simulink model "first"  (R2023b)
settings: Solver=VariableStepAuto  StartTime=0.0  StopTime=10.0  RelTol=1e-3
libraries: arduinolib x13, arduinosensorlib x4
settings Model: Creator=tjrgu  LastModifiedBy=tjrgu

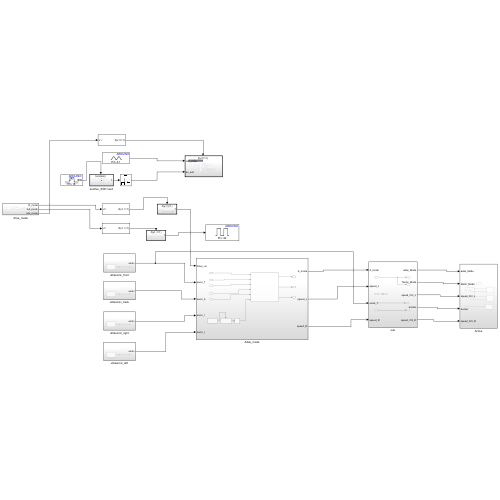
[thumbnail: Simulink's stored preview of the top-level diagram]
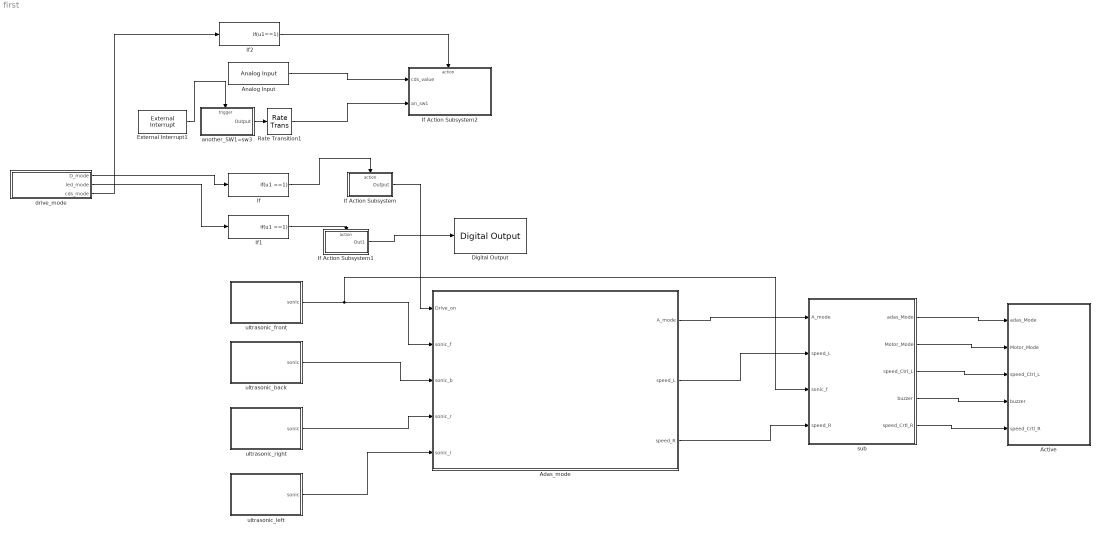
== system first ==
  Active : Subsystem
  Adas_mode : Subsystem
  Analog Input : arduinolib/Analog Input  pinNumber=1  ReadResultsOnly=off  ConversionTriggerSource=Software  ExternalTriggerType=uint32( 0 )  OutputDataType=uint16  EnableConversionCompleteNotify=off  EnableOuputStatus=off  SampleTime=-1  blockPlatform=arduino
  Digital Output : arduinolib/Digital Output  pinNumber=42  Direction=output  blockPlatform=arduino
  External Interrupt1 : arduinolib/External Interrupt  Pin=18  PullUp=off  Mode=RISING  InterruptSimulationInput=off
  If : If  IfExpression=u1 ==1  ShowElse=off
  If Action Subsystem : Subsystem  TreatAsAtomicUnit=on
  If Action Subsystem1 : Subsystem  TreatAsAtomicUnit=on
  If Action Subsystem2 : Subsystem  TreatAsAtomicUnit=on
  If1 : If  IfExpression=u1 ==1  ShowElse=off
  If2 : If  IfExpression=u1==1  ShowElse=off
  Rate Transition1 : RateTransition  Integrity=off
  another_SW1=sw3 : Subsystem
  drive_mode : Subsystem
  sub : Subsystem
  ultrasonic_back : Subsystem
  ultrasonic_front : Subsystem
  ultrasonic_left : Subsystem
  ultrasonic_right : Subsystem
  wires:
  ultrasonic_front/1(sonic) -> sub/3(sonic_f), Adas_mode/2(sonic_f)
  drive_mode/1(D_mode) -> If/1
  ultrasonic_back/1(sonic) -> Adas_mode/3(sonic_b)
  ultrasonic_right/1(sonic) -> Adas_mode/4(sonic_r)
  ultrasonic_left/1(sonic) -> Adas_mode/5(sonic_l)
  Adas_mode/1(A_mode) -> sub/1(A_mode)
  Adas_mode/2(speed_L) -> sub/2(speed_L)
  Adas_mode/3(speed_R) -> sub/4(speed_R)
  sub/1(adas_Mode) -> Active/1(adas_Mode)
  sub/2(Motor_Mode) -> Active/2(Motor_Mode)
  sub/3(speed_Ctrl_L) -> Active/3(speed_Ctrl_L)
  sub/4(buzzer) -> Active/4(buzzer)
  sub/5(speed_Crtl_R) -> Active/5(speed_Crtl_R)
  If/1 -> If Action Subsystem/Action
  If Action Subsystem/1(Output) -> Adas_mode/1(Drive_on)
  drive_mode/2(led_mode) -> If1/1
  If1/1 -> If Action Subsystem1/Action
  If Action Subsystem1/1(Out1) -> Digital Output/1
  drive_mode/3(cds_mode) -> If2/1
  If2/1 -> If Action Subsystem2/Action
  Analog Input/1 -> If Action Subsystem2/1(cds_value)
  External Interrupt1/1 -> another_SW1=sw3/Trigger
  another_SW1=sw3/1(Output) -> Rate Transition1/1
  Rate Transition1/1 -> If Action Subsystem2/2(an_sw1)

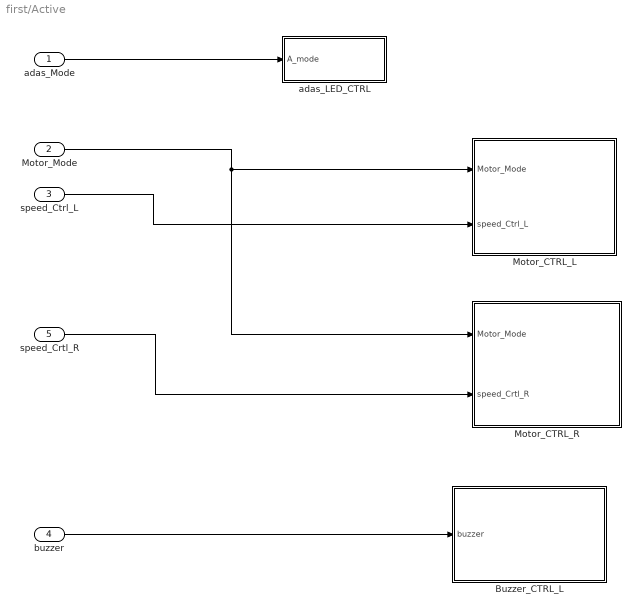
== system first/Active ==
  adas_Mode : Inport
  Motor_Mode : Inport  Port=2
  speed_Ctrl_L : Inport  Port=3
  buzzer : Inport  Port=4
  speed_Crtl_R : Inport  Port=5
  Buzzer_CTRL_L : Subsystem
  Motor_CTRL_L : Subsystem
  Motor_CTRL_R : Subsystem
  adas_LED_CTRL : Subsystem
  wires:
  Motor_Mode/1 -> Motor_CTRL_R/1(Motor_Mode), Motor_CTRL_L/1(Motor_Mode)
  speed_Ctrl_L/1 -> Motor_CTRL_L/2(speed_Ctrl_L)
  speed_Crtl_R/1 -> Motor_CTRL_R/2(speed_Crtl_R)
  buzzer/1 -> Buzzer_CTRL_L/1(buzzer)
  adas_Mode/1 -> adas_LED_CTRL/1(A_mode)

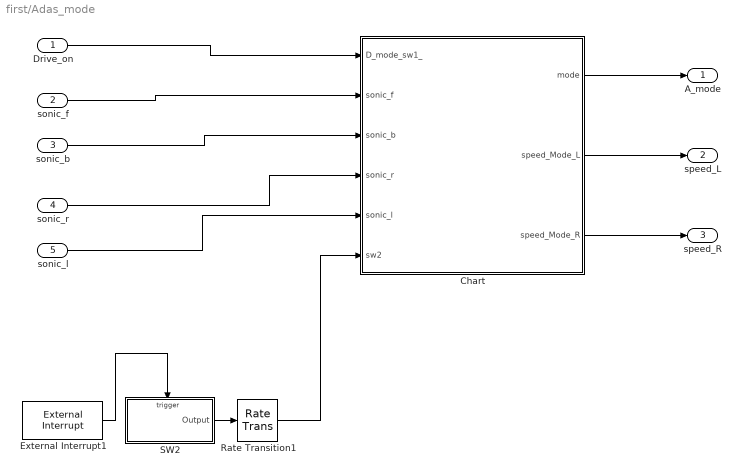
== system first/Adas_mode ==
  Drive_on : Inport
  sonic_f : Inport  Port=2
  sonic_b : Inport  Port=3
  sonic_r : Inport  Port=4
  sonic_l : Inport  Port=5
  Chart : Stateflow chart  TreatAsAtomicUnit=on
  External Interrupt1 : arduinolib/External Interrupt  Pin=3  PullUp=off  Mode=RISING  InterruptSimulationInput=off
  Rate Transition1 : RateTransition  Integrity=off
  SW2 : Subsystem
  A_mode : Outport
  speed_L : Outport  Port=2
  speed_R : Outport  Port=3
  wires:
  sonic_f/1 -> Chart/2(sonic_f)
  External Interrupt1/1 -> SW2/Trigger
  SW2/1(Output) -> Rate Transition1/1
  Rate Transition1/1 -> Chart/6(sw2)
  Drive_on/1 -> Chart/1(D_mode_sw1_)
  sonic_b/1 -> Chart/3(sonic_b)
  sonic_r/1 -> Chart/4(sonic_r)
  sonic_l/1 -> Chart/5(sonic_l)
  Chart/1(mode) -> A_mode/1
  Chart/2(speed_Mode_L) -> speed_L/1
  Chart/3(speed_Mode_R) -> speed_R/1

== system first/If Action Subsystem ==
  Action Port : ActionPort  ActionPortLabel=if(u1 ==1)
  Constant : Constant
  Output : Outport
  wires:
  Constant/1 -> Output/1

== system first/If Action Subsystem1 ==
  Action Port : ActionPort  ActionPortLabel=if(u1 ==1)
  Constant : Constant
  Out1 : Outport
  wires:
  Constant/1 -> Out1/1

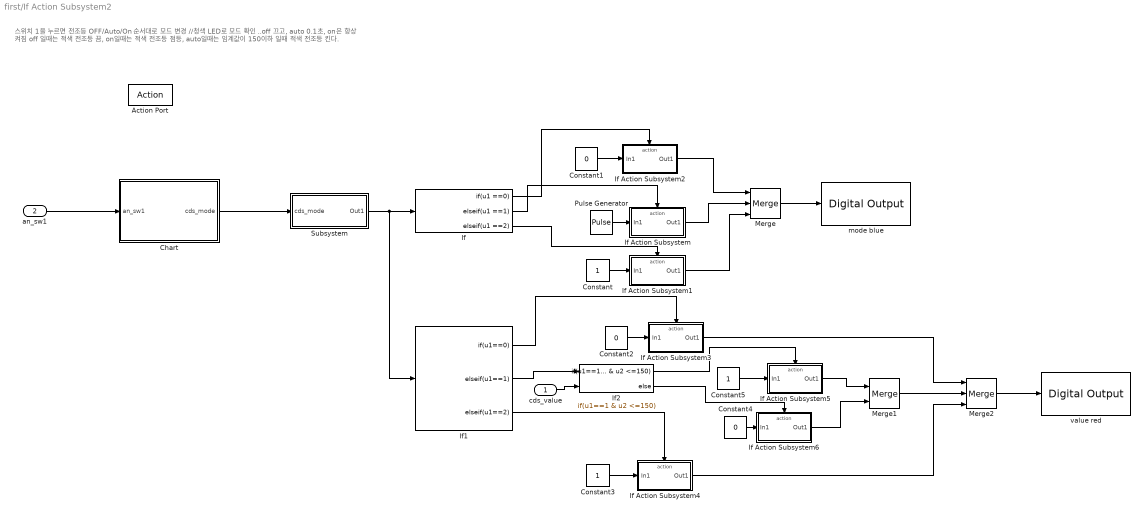
== system first/If Action Subsystem2 ==
  note: 스위치 1을  누르면 전조등 OFF/Auto/On 순서대로 모드 변경 //청색 LED로 모드 확인 ..off 끄고, auto 0.1초, on은 항상 켜짐
      | off 일때는 적색 전조등 끔, on일때는 적색 전조등 점등, auto일때는 임계값이 150이하 일때 적색 전조등 킨다.
  cds_value : Inport
  an_sw1 : Inport  Port=2
  Action Port : ActionPort  ActionPortLabel=if(u1==1)
  Chart : Stateflow chart  TreatAsAtomicUnit=on
  Constant : Constant
  Constant1 : Constant  Value=0
  Constant2 : Constant  Value=0
  Constant3 : Constant
  Constant4 : Constant  Value=0
  Constant5 : Constant
  If : If  IfExpression=u1 ==0  ElseIfExpressions=u1 ==1,u1 ==2  ShowElse=off
  If Action Subsystem : Subsystem  TreatAsAtomicUnit=on
  If Action Subsystem1 : Subsystem  TreatAsAtomicUnit=on
  If Action Subsystem2 : Subsystem  TreatAsAtomicUnit=on
  If Action Subsystem3 : Subsystem  TreatAsAtomicUnit=on
  If Action Subsystem4 : Subsystem  TreatAsAtomicUnit=on
  If Action Subsystem5 : Subsystem  TreatAsAtomicUnit=on
  If Action Subsystem6 : Subsystem  TreatAsAtomicUnit=on
  If1 : If  IfExpression=u1==0  ElseIfExpressions=u1==1, u1==2  ShowElse=off
  If2 : If  NumInputs=2  IfExpression=u1==1 & u2 <=150
  Merge : Merge  Inputs=3
  Merge1 : Merge
  Merge2 : Merge  Inputs=3
  Pulse Generator : DiscretePulseGenerator  PulseType=Time based  Period=0.2  PulseWidth=50
  Subsystem : Subsystem
  mode blue : arduinolib/Digital Output  pinNumber=45  Direction=output  blockPlatform=arduino
  value red : arduinolib/Digital Output  pinNumber=44  Direction=output  blockPlatform=arduino
  wires:
  an_sw1/1 -> Chart/1(an_sw1)
  Chart/1(cds_mode) -> Subsystem/1(cds_mode)
  Subsystem/1(Out1) -> If1/1, If/1
  If/2 -> If Action Subsystem/Action
  Pulse Generator/1 -> If Action Subsystem/1(In1)
  If/3 -> If Action Subsystem1/Action
  Constant/1 -> If Action Subsystem1/1(In1)
  If/1 -> If Action Subsystem2/Action
  Constant1/1 -> If Action Subsystem2/1(In1)
  If Action Subsystem2/1(Out1) -> Merge/1
  If Action Subsystem/1(Out1) -> Merge/2
  If Action Subsystem1/1(Out1) -> Merge/3
  Merge/1 -> mode blue/1
  If1/1 -> If Action Subsystem3/Action
  Constant2/1 -> If Action Subsystem3/1(In1)
  If1/3 -> If Action Subsystem4/Action
  Constant3/1 -> If Action Subsystem4/1(In1)
  If1/2 -> If2/1
  cds_value/1 -> If2/2
  If2/1 -> If Action Subsystem5/Action
  If2/2 -> If Action Subsystem6/Action
  Constant4/1 -> If Action Subsystem6/1(In1)
  Constant5/1 -> If Action Subsystem5/1(In1)
  If Action Subsystem5/1(Out1) -> Merge1/1
  If Action Subsystem6/1(Out1) -> Merge1/2
  If Action Subsystem3/1(Out1) -> Merge2/1
  Merge1/1 -> Merge2/2
  If Action Subsystem4/1(Out1) -> Merge2/3
  Merge2/1 -> value red/1

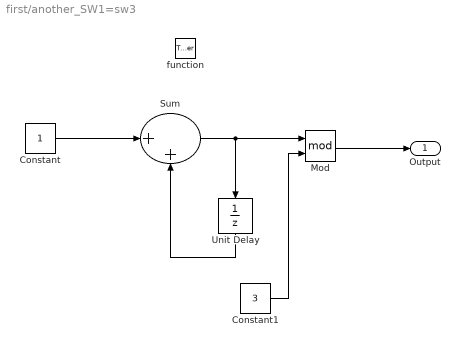
== system first/another_SW1=sw3 ==
  function : TriggerPort  TriggerType=function-call  VariantControl=(inherit)
  Constant : Constant
  Constant1 : Constant  Value=3
  Mod : Math  Operator=mod
  Sum : Sum  Inputs=|++
  Unit Delay : UnitDelay  SampleTime=-1  HasFrameUpgradeWarning=on
  Output : Outport
  wires:
  Constant/1 -> Sum/1
  Sum/1 -> Unit Delay/1, Mod/1
  Constant1/1 -> Mod/2
  Unit Delay/1 -> Sum/2
  Mod/1 -> Output/1

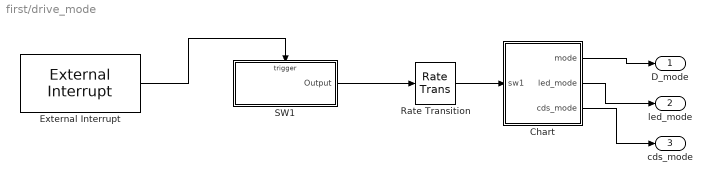
== system first/drive_mode ==
  Chart : Stateflow chart  TreatAsAtomicUnit=on
  External Interrupt : arduinolib/External Interrupt  Pin=2  PullUp=off  Mode=RISING  InterruptSimulationInput=off
  Rate Transition : RateTransition  Integrity=off
  SW1 : Subsystem
  D_mode : Outport
  led_mode : Outport  Port=2
  cds_mode : Outport  Port=3
  wires:
  External Interrupt/1 -> SW1/Trigger
  SW1/1(Output) -> Rate Transition/1
  Rate Transition/1 -> Chart/1(sw1)
  Chart/1(mode) -> D_mode/1
  Chart/2(led_mode) -> led_mode/1
  Chart/3(cds_mode) -> cds_mode/1

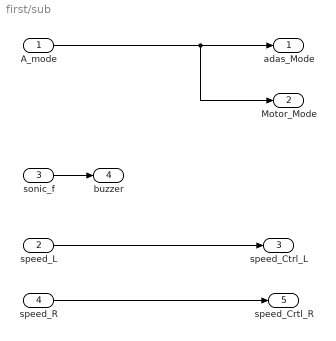
== system first/sub ==
  A_mode : Inport
  speed_L : Inport  Port=2
  sonic_f : Inport  Port=3
  speed_R : Inport  Port=4
  adas_Mode : Outport
  Motor_Mode : Outport  Port=2
  speed_Ctrl_L : Outport  Port=3
  buzzer : Outport  Port=4
  speed_Crtl_R : Outport  Port=5
  wires:
  A_mode/1 -> Motor_Mode/1, adas_Mode/1
  speed_L/1 -> speed_Ctrl_L/1
  speed_R/1 -> speed_Crtl_R/1
  sonic_f/1 -> buzzer/1

== system first/ultrasonic_back ==
  note: 초음파 계수 10
      | 실제 요구사항 : 50cm , 10cm
      | 변경 요구사항 : 초음파값 5,1
  Gain : Gain  Gain=10
  Ultrasonic Sensor : arduinosensorlib/Ultrasonic Sensor  NumSignalPins=2  TrigPin=48  EchoPin=49  SignalPin=3  SampleTime_=0.1  blockPlatform=ARDUINO
  sonic : Outport
  wires:
  Ultrasonic Sensor/1 -> Gain/1
  Gain/1 -> sonic/1

== system first/ultrasonic_front ==
  note: 초음파 계수 10
      | 실제 요구사항 : 50cm , 10cm
      | 변경 요구사항 : 초음파값 5,1
  Gain : Gain  Gain=10
  Ultrasonic Sensor : arduinosensorlib/Ultrasonic Sensor  NumSignalPins=2  TrigPin=46  EchoPin=47  SignalPin=3  SampleTime_=0.1  blockPlatform=ARDUINO
  sonic : Outport
  wires:
  Ultrasonic Sensor/1 -> Gain/1
  Gain/1 -> sonic/1

== system first/ultrasonic_left ==
  note: 초음파 계수 10
      | 실제 요구사항 : 50cm , 10cm
      | 변경 요구사항 : 초음파값 5,1
  Gain : Gain  Gain=10
  Ultrasonic Sensor : arduinosensorlib/Ultrasonic Sensor  NumSignalPins=2  TrigPin=52  EchoPin=53  SignalPin=3  SampleTime_=0.1  blockPlatform=ARDUINO
  sonic : Outport
  wires:
  Ultrasonic Sensor/1 -> Gain/1
  Gain/1 -> sonic/1

== system first/ultrasonic_right ==
  note: 초음파 계수 10
      | 실제 요구사항 : 50cm , 10cm
      | 변경 요구사항 : 초음파값 5,1
  Gain : Gain  Gain=10
  Ultrasonic Sensor : arduinosensorlib/Ultrasonic Sensor  NumSignalPins=2  TrigPin=50  EchoPin=51  SignalPin=3  SampleTime_=0.1  blockPlatform=ARDUINO
  sonic : Outport
  wires:
  Ultrasonic Sensor/1 -> Gain/1
  Gain/1 -> sonic/1

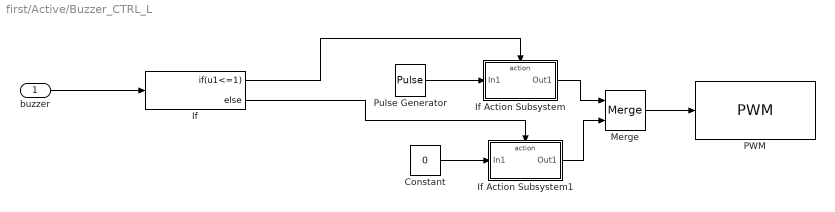
== system first/Active/Buzzer_CTRL_L ==
  buzzer : Inport
  Constant : Constant  Value=0
  If : If  IfExpression=u1<=1
  If Action Subsystem : Subsystem  TreatAsAtomicUnit=on
  If Action Subsystem1 : Subsystem  TreatAsAtomicUnit=on
  Merge : Merge
  PWM : arduinolib/PWM  pinNumber=4  frequencyType=Default  desiredFrequency=490.2  achievableFrequency=490.2
  Pulse Generator : DiscretePulseGenerator  PulseType=Time based  Period=0.4  PulseWidth=50
  wires:
  buzzer/1 -> If/1
  Pulse Generator/1 -> If Action Subsystem/1(In1)
  If/2 -> If Action Subsystem1/Action
  Constant/1 -> If Action Subsystem1/1(In1)
  If Action Subsystem/1(Out1) -> Merge/1
  If Action Subsystem1/1(Out1) -> Merge/2
  Merge/1 -> PWM/1
  If/1 -> If Action Subsystem/Action

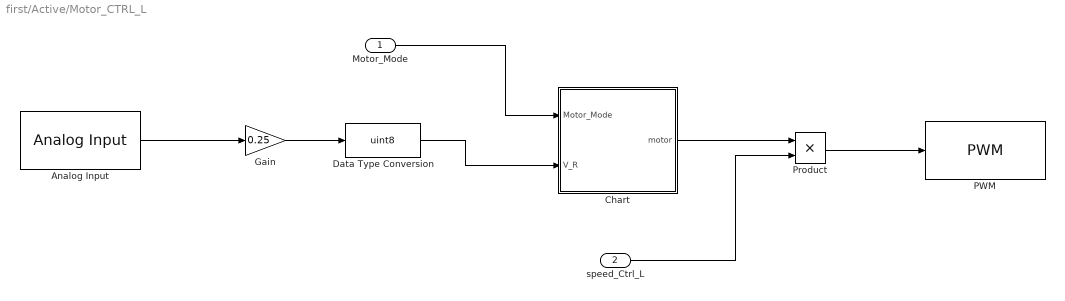
== system first/Active/Motor_CTRL_L ==
  Motor_Mode : Inport
  speed_Ctrl_L : Inport  Port=2
  Analog Input : arduinolib/Analog Input  pinNumber=0  ReadResultsOnly=off  ConversionTriggerSource=Software  ExternalTriggerType=uint32( 0 )  OutputDataType=uint16  EnableConversionCompleteNotify=off  EnableOuputStatus=off  SampleTime=-1  blockPlatform=arduino
  Chart : Stateflow chart  TreatAsAtomicUnit=on
  Data Type Conversion : DataTypeConversion  OutDataTypeStr=uint8  SaturateOnIntegerOverflow=off  RndMeth=Floor
  Gain : Gain  Gain=0.25
  PWM : arduinolib/PWM  pinNumber=11  frequencyType=Default  desiredFrequency=490.2  achievableFrequency=490.2
  Product : Product
  wires:
  Analog Input/1 -> Gain/1
  Gain/1 -> Data Type Conversion/1
  Motor_Mode/1 -> Chart/1(Motor_Mode)
  Data Type Conversion/1 -> Chart/2(V_R)
  Chart/1(motor) -> Product/1
  speed_Ctrl_L/1 -> Product/2
  Product/1 -> PWM/1

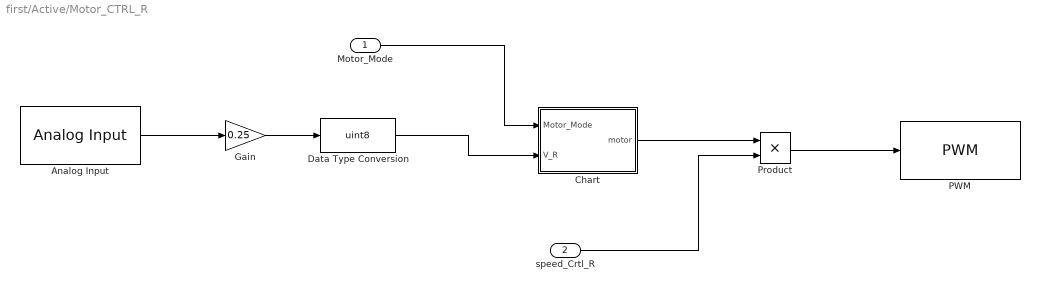
== system first/Active/Motor_CTRL_R ==
  Motor_Mode : Inport
  speed_Crtl_R : Inport  Port=2
  Analog Input : arduinolib/Analog Input  pinNumber=0  ReadResultsOnly=off  ConversionTriggerSource=Software  ExternalTriggerType=uint32( 0 )  OutputDataType=uint16  EnableConversionCompleteNotify=off  EnableOuputStatus=off  SampleTime=-1  blockPlatform=arduino
  Chart : Stateflow chart  TreatAsAtomicUnit=on
  Data Type Conversion : DataTypeConversion  OutDataTypeStr=uint8  SaturateOnIntegerOverflow=off  RndMeth=Floor
  Gain : Gain  Gain=0.25
  PWM : arduinolib/PWM  pinNumber=3  frequencyType=Default  desiredFrequency=490.2  achievableFrequency=490.2
  Product : Product
  wires:
  Gain/1 -> Data Type Conversion/1
  Analog Input/1 -> Gain/1
  Motor_Mode/1 -> Chart/1(Motor_Mode)
  Data Type Conversion/1 -> Chart/2(V_R)
  Chart/1(motor) -> Product/1
  speed_Crtl_R/1 -> Product/2
  Product/1 -> PWM/1

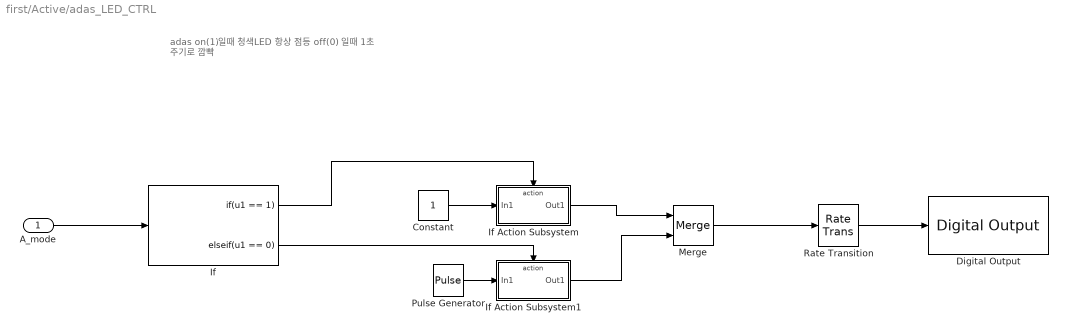
== system first/Active/adas_LED_CTRL ==
  note: adas on(1)일때 청색LED 항상 점등
      | off(0) 일때 1초 주기로 깜빡
  A_mode : Inport
  Constant : Constant
  Digital Output : arduinolib/Digital Output  pinNumber=43  Direction=output  blockPlatform=arduino
  If : If  IfExpression=u1 == 1  ElseIfExpressions=u1 == 0  ShowElse=off
  If Action Subsystem : Subsystem  TreatAsAtomicUnit=on
  If Action Subsystem1 : Subsystem  TreatAsAtomicUnit=on
  Merge : Merge
  Pulse Generator : DiscretePulseGenerator  PulseType=Time based  PulseWidth=50
  Rate Transition : RateTransition  Integrity=off
  wires:
  A_mode/1 -> If/1
  If/1 -> If Action Subsystem/Action
  Constant/1 -> If Action Subsystem/1(In1)
  If/2 -> If Action Subsystem1/Action
  Pulse Generator/1 -> If Action Subsystem1/1(In1)
  If Action Subsystem/1(Out1) -> Merge/1
  If Action Subsystem1/1(Out1) -> Merge/2
  Merge/1 -> Rate Transition/1
  Rate Transition/1 -> Digital Output/1

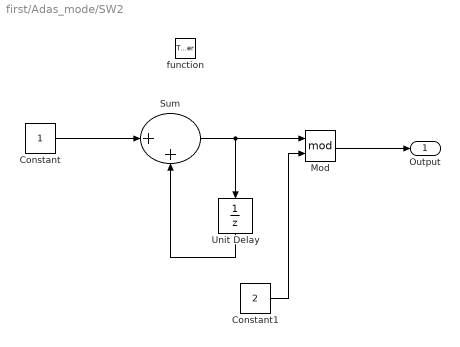
== system first/Adas_mode/SW2 ==
  function : TriggerPort  TriggerType=function-call  VariantControl=(inherit)
  Constant : Constant
  Constant1 : Constant  Value=2
  Mod : Math  Operator=mod
  Sum : Sum  Inputs=|++
  Unit Delay : UnitDelay  SampleTime=-1  HasFrameUpgradeWarning=on
  Output : Outport
  wires:
  Constant/1 -> Sum/1
  Sum/1 -> Unit Delay/1, Mod/1
  Constant1/1 -> Mod/2
  Unit Delay/1 -> Sum/2
  Mod/1 -> Output/1

== system first/If Action Subsystem2/If Action Subsystem ==
  In1 : Inport
  Action Port : ActionPort  ActionPortLabel=elseif(u1 ==1)
  Out1 : Outport
  wires:
  In1/1 -> Out1/1

== system first/If Action Subsystem2/If Action Subsystem1 ==
  In1 : Inport
  Action Port : ActionPort  ActionPortLabel=elseif(u1 ==2)
  Out1 : Outport
  wires:
  In1/1 -> Out1/1

== system first/If Action Subsystem2/If Action Subsystem2 ==
  In1 : Inport
  Action Port : ActionPort  ActionPortLabel=if(u1 ==0)
  Out1 : Outport
  wires:
  In1/1 -> Out1/1

== system first/If Action Subsystem2/If Action Subsystem3 ==
  In1 : Inport
  Action Port : ActionPort  ActionPortLabel=if(u1==0)
  Out1 : Outport
  wires:
  In1/1 -> Out1/1

== system first/If Action Subsystem2/If Action Subsystem4 ==
  In1 : Inport
  Action Port : ActionPort  ActionPortLabel=elseif( u1==2)
  Out1 : Outport
  wires:
  In1/1 -> Out1/1

== system first/If Action Subsystem2/If Action Subsystem5 ==
  In1 : Inport
  Action Port : ActionPort  ActionPortLabel=if(u1==1 & u2 <=150)
  Out1 : Outport
  wires:
  In1/1 -> Out1/1

== system first/If Action Subsystem2/If Action Subsystem6 ==
  In1 : Inport
  Action Port : ActionPort  ActionPortLabel=else
  Out1 : Outport
  wires:
  In1/1 -> Out1/1

== system first/If Action Subsystem2/Subsystem ==
  cds_mode : Inport
  Out1 : Outport
  wires:
  cds_mode/1 -> Out1/1

== system first/drive_mode/SW1 ==
  function : TriggerPort  TriggerType=function-call  VariantControl=(inherit)
  Constant : Constant
  Constant1 : Constant  Value=2
  Mod : Math  Operator=mod
  Sum : Sum  Inputs=|++
  Unit Delay : UnitDelay  SampleTime=-1  HasFrameUpgradeWarning=on
  Output : Outport
  wires:
  Constant/1 -> Sum/1
  Sum/1 -> Unit Delay/1, Mod/1
  Constant1/1 -> Mod/2
  Unit Delay/1 -> Sum/2
  Mod/1 -> Output/1

== system first/Active/Buzzer_CTRL_L/If Action Subsystem ==
  In1 : Inport
  Action Port : ActionPort  ActionPortLabel=if(u1<=1)
  Out1 : Outport
  wires:
  In1/1 -> Out1/1

== system first/Active/Buzzer_CTRL_L/If Action Subsystem1 ==
  In1 : Inport
  Action Port : ActionPort  ActionPortLabel=else
  Out1 : Outport
  wires:
  In1/1 -> Out1/1

== system first/Active/adas_LED_CTRL/If Action Subsystem ==
  In1 : Inport
  Action Port : ActionPort  ActionPortLabel=if(u1 == 0)
  Out1 : Outport
  wires:
  In1/1 -> Out1/1

== system first/Active/adas_LED_CTRL/If Action Subsystem1 ==
  In1 : Inport
  Action Port : ActionPort  ActionPortLabel=elseif(u1 == 1)
  Out1 : Outport
  wires:
  In1/1 -> Out1/1

== stateflow chart first/Adas_mode/Chart ==
  state Drive_on_ 상태 [group]
    adas on/off 기능
  state adas_On_stop %전방 10cm 이내
    en, du:
    speed_Mode_L =0;
    speed_Mode_R = 0;
    mode = sw2;
    state_2 = sw2;
  state Left_control
  state adas_on
    en,du:
    mode = sw2;
    speed_Mode_L =1;
    speed_Mode_R=1;
    state_2 =sw2;
  state adas_off
    en,du:
    mode = sw2;
    speed_Mode_L =1;
    speed_Mode_R =1;
    state_2 = sw2;
  state Right_control2
  state adas_On_increase %후방 10cm 이내
    en,du:
    speed_Mode_L = 1.2;
    speed_Mode_R = 1.2;
    mode =sw2;
    state_2 = sw2;
  adas_on -> adas_On_stop %전방 10cm 이내 [order 3] : [sonic_f <=1]
  adas_On_stop %전방 10cm 이내 -> adas_on : [sonic_f >1]
  adas_on -> adas_On_stop %전방 10cm 이내 [order 4] : [sonic_f <=1 && sonic_b <=1 ]
  (default) -> adas_off
  adas_off -> adas_on : [state_2 ~= sw2]
  adas_on -> adas_off [order 1] : [state_2 ~= sw2]
  adas_on -> adas_On_increase %후방 10cm 이내 [order 2] : [sonic_b <= 1]
  adas_On_increase %후방 10cm 이내 -> adas_on : [sonic_b >1]
  data: D_mode_sw1_ input; sonic_f input; sonic_b input; sonic_r input; sonic_l input; sw2 input; mode output; speed_Mode_L output; speed_Mode_R output; state_2 local

== stateflow chart first/Active/Motor_CTRL_L/Chart ==
  state adas_off
    en,du:
    motor = 0;
  state adas_on
    en:
    speed = V_R;
    du:
    motor = speed;
  (default) -> adas_off
  adas_off -> adas_on : [Motor_Mode ==1 ]
  adas_on -> adas_off : [Motor_Mode == 0]
  data: Motor_Mode input; V_R input; motor output; speed local

== stateflow chart first/drive_mode/Chart ==
  state acc_off
    en, du:
    mode = sw1;
    led_mode = sw1;
    cds_mode = sw1;
    %speed_Mode =1;
    state_1 = sw1;
  state acc_on
    en,du:
    mode =sw1;
    led_mode =sw1;
    cds_mode = sw1;
    %speed_Mode =1;
    state_1 = sw1;
  (default) -> acc_off
  acc_off -> acc_on : [state_1 ~= sw1]
  acc_on -> acc_off : [state_1~=sw1]
  data: sw1 input; mode output; state_1 local; led_mode output; cds_mode output

== stateflow chart first/Active/Motor_CTRL_R/Chart ==
  state adas_off
    en,du:
    motor = 0;
  state adas_on
    en:
    speed = V_R;
    du:
    motor = speed;
  (default) -> adas_off
  adas_off -> adas_on : [Motor_Mode ==1 ]
  adas_on -> adas_off : [Motor_Mode == 0]
  data: Motor_Mode input; V_R input; motor output; speed local

== stateflow chart first/If Action Subsystem2/Chart ==
  state cds_auto
    en, du:
    %led_mode = an_sw1;
    cds_mode = an_sw1;
    state_1 = an_sw1;
  state cds_off
    en, du:
    %led_mode = an_sw1;
    cds_mode =an_sw1;
    state_1 = an_sw1;
  state cds_on
    en,du:
    % led_mode = an_sw1;
    cds_mode =an_sw1;
    state_1 = an_sw1;
  cds_auto -> cds_on : [state_1 ~= an_sw1]
  cds_off -> cds_auto [order 2] : [state_1~=an_sw1]
  (default) -> cds_off
  cds_off -> cds_on [order 1] : [state_1 ~= an_sw1]
  data: an_sw1 input; state_1 local; cds_mode output
